simulink library "goose_lib"  (Simulink 8.1)
settings: Solver=ode45  StartTime=0.0  StopTime=10.0  RelTol=1e-3
undefined symbols (not defined in the file or in its folder): CD, relay_iec61850
libraries: rtio_iec61850 x53
settings Model: Creator=re25624  LastModifiedBy=hptb1

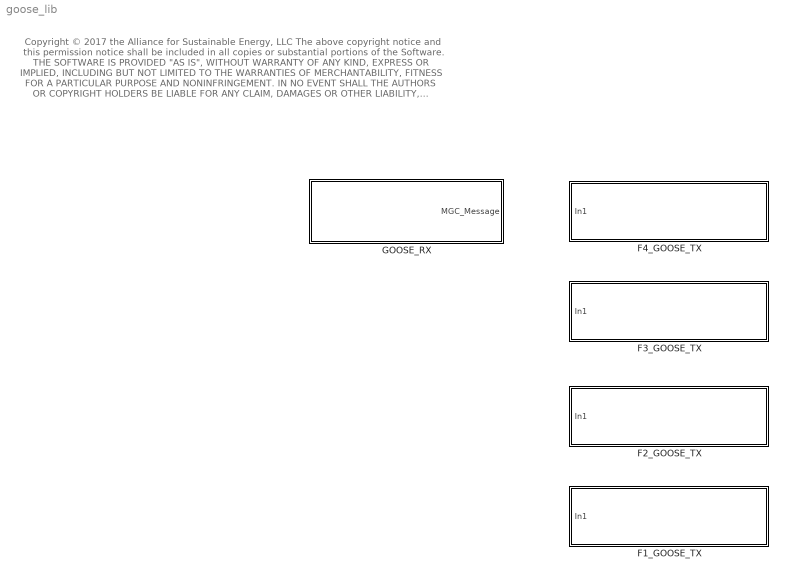
== system goose_lib ==
  note: Copyright © 2017 the Alliance for Sustainable Energy, LLC
      |
      | The above copyright notice and this permission notice shall be included in all copies or substantial portions of the Software.
      |
      | THE SOFTWARE IS PROVIDED "AS IS", WITHOUT WARRANTY OF ANY KIND, EXPRESS OR IMPLIED, INCLUDING
      | BUT NOT LIMITED TO THE WARRANTIES OF MERCHANTABILITY, FITNESS FOR A PARTICULAR PURPOSE AND
      | NONINFRINGEMENT. IN NO EVENT SHALL THE AUTHORS OR COPYRIGHT HOLDERS BE LIABLE FOR ANY CLAIM,
      |  DAMAGES OR OTHER LIABILITY, WHETHER IN AN ACTION OF CONTRACT, TORT OR OTHERWISE, ARISING FROM,
      | OUT OF OR IN CONNECTION WITH THE SOFTWARE OR THE USE OR OTHER DEALINGS IN THE SOFTWARE
  F1_GOOSE_TX : Subsystem
  F2_GOOSE_TX : Subsystem
  F3_GOOSE_TX : Subsystem
  F4_GOOSE_TX : Subsystem
  "GOOSE_RX " : Subsystem

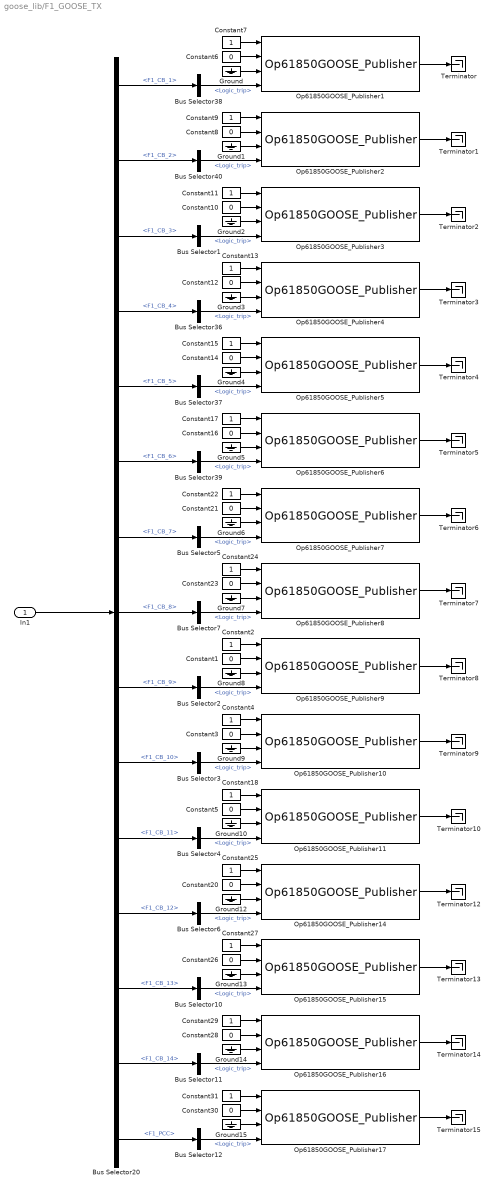
== system goose_lib/F1_GOOSE_TX ==
  In1 : Inport
  Bus Selector{1..7,10..12,36..40} (15 alike) : BusSelector  OutputSignals=Logic_trip
  Bus Selector20 : BusSelector  OutputSignals=F1_CB_1,F1_CB_2,F1_CB_3,F1_CB_4,F1_CB_5,F1_CB_6,F1_CB_7,F1_CB_8,F1_CB_9,F1_CB_10,F1_CB_11,F1_CB_12,F1_CB_13,F1_CB_14,F1_PCC
  Constant{1,3,5..6,8,10,12,14,16,20..21,23,26,28,30} (15 alike) : Constant  Value=0
  Constant{2,4,7,9,11,13,15,17..18,22,24..25,27,29,31} (15 alike) : Constant
  Ground{,1..10,12..15} (15 alike) : Ground
  Op61850GOOSE_Publisher1 : rtio_iec61850/Op61850GOOSE_Publisher  nic_name=eth1  ied_name=CB101  select_scl=off  scl_file=CB101.icd  scl_fullpath=.\relay_iec61850  goose_name=Goose_TRIP1  goose_msgid=0x0101  mac_address=01-0C-CD-01-21-01  vlan_prio=4  vlan_id=000  mintime=25  maxtime=250  gocbref=CB101LDevice1/LLN0$GO$CB_Goose_TRIP1  dataset=CB101LDevice1/LLN0$Goose_TRIP1  goID=Goose_TRIP1  confrev=1  externalClock=off
      settings: AttributesFormatString=%<Name>\nAppId = %<goose_msgid>
  Op61850GOOSE_Publisher10 : rtio_iec61850/Op61850GOOSE_Publisher  nic_name=eth1  ied_name=CB110  select_scl=off  scl_file=CB110.icd  scl_fullpath=.\relay_iec61850  goose_name=Goose_TRIP1  goose_msgid=0x0110  mac_address=01-0C-CD-01-21-10  vlan_prio=4  vlan_id=000  mintime=25  maxtime=250  gocbref=CB110LDevice1/LLN0$GO$CB_Goose_TRIP1  dataset=CB110LDevice1/LLN0$Goose_TRIP1  goID=Goose_TRIP1  confrev=1  externalClock=off
      settings: AttributesFormatString=%<Name>\nAppId = %<goose_msgid>
  Op61850GOOSE_Publisher11 : rtio_iec61850/Op61850GOOSE_Publisher  nic_name=eth1  ied_name=CB111  select_scl=off  scl_file=CB111.icd  scl_fullpath=.\relay_iec61850  goose_name=Goose_TRIP1  goose_msgid=0x0111  mac_address=01-0C-CD-01-21-11  vlan_prio=4  vlan_id=000  mintime=25  maxtime=250  gocbref=CB111LDevice1/LLN0$GO$CB_Goose_TRIP1  dataset=CB111LDevice1/LLN0$Goose_TRIP1  goID=Goose_TRIP1  confrev=1  externalClock=off
      settings: AttributesFormatString=%<Name>\nAppId = %<goose_msgid>
  Op61850GOOSE_Publisher14 : rtio_iec61850/Op61850GOOSE_Publisher  nic_name=eth1  ied_name=CB112  select_scl=off  scl_file=CB112.icd  scl_fullpath=.\relay_iec61850  goose_name=Goose_TRIP1  goose_msgid=0x0112  mac_address=01-0C-CD-01-21-12  vlan_prio=4  vlan_id=000  mintime=25  maxtime=250  gocbref=CB112LDevice1/LLN0$GO$CB_Goose_TRIP1  dataset=CB112LDevice1/LLN0$Goose_TRIP1  goID=Goose_TRIP1  confrev=1  externalClock=off
      settings: AttributesFormatString=%<Name>\nAppId = %<goose_msgid>
  Op61850GOOSE_Publisher15 : rtio_iec61850/Op61850GOOSE_Publisher  nic_name=eth1  ied_name=CB113  select_scl=off  scl_file=CB113.icd  scl_fullpath=.\relay_iec61850  goose_name=Goose_TRIP1  goose_msgid=0x0113  mac_address=01-0C-CD-01-21-13  vlan_prio=4  vlan_id=000  mintime=25  maxtime=250  gocbref=CB113LDevice1/LLN0$GO$CB_Goose_TRIP1  dataset=CB113LDevice1/LLN0$Goose_TRIP1  goID=Goose_TRIP1  confrev=1  externalClock=off
      settings: AttributesFormatString=%<Name>\nAppId = %<goose_msgid>
  Op61850GOOSE_Publisher16 : rtio_iec61850/Op61850GOOSE_Publisher  nic_name=eth1  ied_name=CB114  select_scl=off  scl_file=CB114.icd  scl_fullpath=.\relay_iec61850  goose_name=Goose_TRIP1  goose_msgid=0x0114  mac_address=01-0C-CD-01-21-14  vlan_prio=4  vlan_id=000  mintime=25  maxtime=250  gocbref=CB114LDevice1/LLN0$GO$CB_Goose_TRIP1  dataset=CB114LDevice1/LLN0$Goose_TRIP1  goID=Goose_TRIP1  confrev=1  externalClock=off
      settings: AttributesFormatString=%<Name>\nAppId = %<goose_msgid>
  Op61850GOOSE_Publisher17 : rtio_iec61850/Op61850GOOSE_Publisher  nic_name=eth1  ied_name=CB100  select_scl=off  scl_file=CB100.icd  scl_fullpath=.\relay_iec61850  goose_name=Goose_TRIP1  goose_msgid=0x0100  mac_address=01-0C-CD-01-21-00  vlan_prio=4  vlan_id=000  mintime=25  maxtime=250  gocbref=CB100LDevice1/LLN0$GO$CB_Goose_TRIP1  dataset=CB100LDevice1/LLN0$Goose_TRIP1  goID=Goose_TRIP1  confrev=1  externalClock=off
      settings: AttributesFormatString=%<Name>\nAppId = %<goose_msgid>
  Op61850GOOSE_Publisher2 : rtio_iec61850/Op61850GOOSE_Publisher  nic_name=eth1  ied_name=CB102  select_scl=off  scl_file=CB102.icd  scl_fullpath=.\relay_iec61850  goose_name=Goose_TRIP1  goose_msgid=0x0102  mac_address=01-0C-CD-01-21-02  vlan_prio=4  vlan_id=000  mintime=25  maxtime=250  gocbref=CB102LDevice1/LLN0$GO$CB_Goose_TRIP1  dataset=CB102LDevice1/LLN0$Goose_TRIP1  goID=Goose_TRIP1  confrev=1  externalClock=off
      settings: AttributesFormatString=%<Name>\nAppId = %<goose_msgid>
  Op61850GOOSE_Publisher3 : rtio_iec61850/Op61850GOOSE_Publisher  nic_name=eth1  ied_name=CB103  select_scl=off  scl_file=CB103.icd  scl_fullpath=.\relay_iec61850  goose_name=Goose_TRIP1  goose_msgid=0x0103  mac_address=01-0C-CD-01-21-03  vlan_prio=4  vlan_id=000  mintime=25  maxtime=250  gocbref=CB103LDevice1/LLN0$GO$CB_Goose_TRIP1  dataset=CB103LDevice1/LLN0$Goose_TRIP1  goID=Goose_TRIP1  confrev=1  externalClock=off
      settings: AttributesFormatString=%<Name>\nAppId = %<goose_msgid>
  Op61850GOOSE_Publisher4 : rtio_iec61850/Op61850GOOSE_Publisher  nic_name=eth1  ied_name=CB104  select_scl=off  scl_file=CB104.icd  scl_fullpath=.\relay_iec61850  goose_name=Goose_TRIP1  goose_msgid=0x0104  mac_address=01-0C-CD-01-21-04  vlan_prio=4  vlan_id=000  mintime=25  maxtime=250  gocbref=CB104LDevice1/LLN0$GO$CB_Goose_TRIP1  dataset=CB104LDevice1/LLN0$Goose_TRIP1  goID=Goose_TRIP1  confrev=1  externalClock=off
      settings: AttributesFormatString=%<Name>\nAppId = %<goose_msgid>
  Op61850GOOSE_Publisher5 : rtio_iec61850/Op61850GOOSE_Publisher  nic_name=eth1  ied_name=CB105  select_scl=off  scl_file=CB105.icd  scl_fullpath=.\relay_iec61850  goose_name=Goose_TRIP1  goose_msgid=0x0105  mac_address=01-0C-CD-01-21-05  vlan_prio=4  vlan_id=000  mintime=25  maxtime=250  gocbref=CB105LDevice1/LLN0$GO$CB_Goose_TRIP1  dataset=CB105LDevice1/LLN0$Goose_TRIP1  goID=Goose_TRIP1  confrev=1  externalClock=off
      settings: AttributesFormatString=%<Name>\nAppId = %<goose_msgid>
  Op61850GOOSE_Publisher6 : rtio_iec61850/Op61850GOOSE_Publisher  nic_name=eth1  ied_name=CB106  select_scl=off  scl_file=CB106.icd  scl_fullpath=.\relay_iec61850  goose_name=Goose_TRIP1  goose_msgid=0x0106  mac_address=01-0C-CD-01-21-06  vlan_prio=4  vlan_id=000  mintime=25  maxtime=250  gocbref=CB106LDevice1/LLN0$GO$CB_Goose_TRIP1  dataset=CB106LDevice1/LLN0$Goose_TRIP1  goID=Goose_TRIP1  confrev=1  externalClock=off
      settings: AttributesFormatString=%<Name>\nAppId = %<goose_msgid>
  Op61850GOOSE_Publisher7 : rtio_iec61850/Op61850GOOSE_Publisher  nic_name=eth1  ied_name=CB107  select_scl=off  scl_file=CB107.icd  scl_fullpath=.\relay_iec61850  goose_name=Goose_TRIP1  goose_msgid=0x0107  mac_address=01-0C-CD-01-21-07  vlan_prio=4  vlan_id=000  mintime=25  maxtime=250  gocbref=CB107LDevice1/LLN0$GO$CB_Goose_TRIP1  dataset=CB107LDevice1/LLN0$Goose_TRIP1  goID=Goose_TRIP1  confrev=1  externalClock=off
      settings: AttributesFormatString=%<Name>\nAppId = %<goose_msgid>
  Op61850GOOSE_Publisher8 : rtio_iec61850/Op61850GOOSE_Publisher  nic_name=eth1  ied_name=CB108  select_scl=off  scl_file=CB108.icd  scl_fullpath=.\relay_iec61850  goose_name=Goose_TRIP1  goose_msgid=0x0108  mac_address=01-0C-CD-01-21-08  vlan_prio=4  vlan_id=000  mintime=25  maxtime=250  gocbref=CB108LDevice1/LLN0$GO$CB_Goose_TRIP1  dataset=CB108LDevice1/LLN0$Goose_TRIP1  goID=Goose_TRIP1  confrev=1  externalClock=off
      settings: AttributesFormatString=%<Name>\nAppId = %<goose_msgid>
  Op61850GOOSE_Publisher9 : rtio_iec61850/Op61850GOOSE_Publisher  nic_name=eth1  ied_name=CB109  select_scl=off  scl_file=CB109.icd  scl_fullpath=.\relay_iec61850  goose_name=Goose_TRIP1  goose_msgid=0x0109  mac_address=01-0C-CD-01-21-09  vlan_prio=4  vlan_id=000  mintime=25  maxtime=250  gocbref=CB109LDevice1/LLN0$GO$CB_Goose_TRIP1  dataset=CB109LDevice1/LLN0$Goose_TRIP1  goID=Goose_TRIP1  confrev=1  externalClock=off
      settings: AttributesFormatString=%<Name>\nAppId = %<goose_msgid>
  Terminator{,1..10,12..15} (15 alike) : Terminator
  wires:
  Ground15/1 -> Op61850GOOSE_Publisher17/3
  Constant31/1 -> Op61850GOOSE_Publisher17/1
  Ground13/1 -> Op61850GOOSE_Publisher15/3
  Constant30/1 -> Op61850GOOSE_Publisher17/2
  Bus Selector12/1 -> Op61850GOOSE_Publisher17/4  "<Logic_trip>"
  Bus Selector20/15 -> Bus Selector12/1  "<F1_PCC>"
  Op61850GOOSE_Publisher16/1 -> Terminator14/1
  Ground14/1 -> Op61850GOOSE_Publisher16/3
  Constant26/1 -> Op61850GOOSE_Publisher15/2
  Constant27/1 -> Op61850GOOSE_Publisher15/1
  Bus Selector10/1 -> Op61850GOOSE_Publisher15/4  "<Logic_trip>"
  Bus Selector20/13 -> Bus Selector10/1  "<F1_CB_13>"
  Op61850GOOSE_Publisher14/1 -> Terminator12/1
  Ground12/1 -> Op61850GOOSE_Publisher14/3
  Op61850GOOSE_Publisher15/1 -> Terminator13/1
  Constant28/1 -> Op61850GOOSE_Publisher16/2
  Constant25/1 -> Op61850GOOSE_Publisher14/1
  Constant20/1 -> Op61850GOOSE_Publisher14/2
  Constant29/1 -> Op61850GOOSE_Publisher16/1
  Bus Selector11/1 -> Op61850GOOSE_Publisher16/4  "<Logic_trip>"
  Bus Selector20/14 -> Bus Selector11/1  "<F1_CB_14>"
  Bus Selector20/12 -> Bus Selector6/1  "<F1_CB_12>"
  Bus Selector6/1 -> Op61850GOOSE_Publisher14/4  "<Logic_trip>"
  Op61850GOOSE_Publisher17/1 -> Terminator15/1
  Ground5/1 -> Op61850GOOSE_Publisher6/3
  Constant17/1 -> Op61850GOOSE_Publisher6/1
  Ground3/1 -> Op61850GOOSE_Publisher4/3
  Ground1/1 -> Op61850GOOSE_Publisher2/3
  In1/1 -> Bus Selector20/1
  Constant16/1 -> Op61850GOOSE_Publisher6/2
  Bus Selector39/1 -> Op61850GOOSE_Publisher6/4  "<Logic_trip>"
  Bus Selector20/6 -> Bus Selector39/1  "<F1_CB_6>"
  Op61850GOOSE_Publisher5/1 -> Terminator4/1
  Ground4/1 -> Op61850GOOSE_Publisher5/3
  Constant12/1 -> Op61850GOOSE_Publisher4/2
  Constant13/1 -> Op61850GOOSE_Publisher4/1
  Bus Selector36/1 -> Op61850GOOSE_Publisher4/4  "<Logic_trip>"
  Bus Selector20/4 -> Bus Selector36/1  "<F1_CB_4>"
  Op61850GOOSE_Publisher3/1 -> Terminator2/1
  Constant9/1 -> Op61850GOOSE_Publisher2/1
  Constant8/1 -> Op61850GOOSE_Publisher2/2
  Bus Selector40/1 -> Op61850GOOSE_Publisher2/4  "<Logic_trip>"
  Bus Selector20/2 -> Bus Selector40/1  "<F1_CB_2>"
  Ground2/1 -> Op61850GOOSE_Publisher3/3
  Op61850GOOSE_Publisher1/1 -> Terminator/1
  Op61850GOOSE_Publisher2/1 -> Terminator1/1
  Op61850GOOSE_Publisher4/1 -> Terminator3/1
  Constant14/1 -> Op61850GOOSE_Publisher5/2
  Constant7/1 -> Op61850GOOSE_Publisher1/1
  Ground/1 -> Op61850GOOSE_Publisher1/3
  Constant11/1 -> Op61850GOOSE_Publisher3/1
  Constant10/1 -> Op61850GOOSE_Publisher3/2
  Constant15/1 -> Op61850GOOSE_Publisher5/1
  Bus Selector37/1 -> Op61850GOOSE_Publisher5/4  "<Logic_trip>"
  Bus Selector20/5 -> Bus Selector37/1  "<F1_CB_5>"
  Bus Selector38/1 -> Op61850GOOSE_Publisher1/4  "<Logic_trip>"
  Bus Selector20/1 -> Bus Selector38/1  "<F1_CB_1>"
  Bus Selector20/3 -> Bus Selector1/1  "<F1_CB_3>"
  Bus Selector1/1 -> Op61850GOOSE_Publisher3/4  "<Logic_trip>"
  Constant6/1 -> Op61850GOOSE_Publisher1/2
  Op61850GOOSE_Publisher6/1 -> Terminator5/1
  Ground9/1 -> Op61850GOOSE_Publisher10/3
  Ground7/1 -> Op61850GOOSE_Publisher8/3
  Op61850GOOSE_Publisher11/1 -> Terminator10/1
  Ground10/1 -> Op61850GOOSE_Publisher11/3
  Constant3/1 -> Op61850GOOSE_Publisher10/2
  Constant4/1 -> Op61850GOOSE_Publisher10/1
  Bus Selector3/1 -> Op61850GOOSE_Publisher10/4  "<Logic_trip>"
  Op61850GOOSE_Publisher9/1 -> Terminator8/1
  Constant24/1 -> Op61850GOOSE_Publisher8/1
  Constant23/1 -> Op61850GOOSE_Publisher8/2
  Bus Selector7/1 -> Op61850GOOSE_Publisher8/4  "<Logic_trip>"
  Ground8/1 -> Op61850GOOSE_Publisher9/3
  Op61850GOOSE_Publisher7/1 -> Terminator6/1
  Op61850GOOSE_Publisher8/1 -> Terminator7/1
  Op61850GOOSE_Publisher10/1 -> Terminator9/1
  Constant5/1 -> Op61850GOOSE_Publisher11/2
  Constant22/1 -> Op61850GOOSE_Publisher7/1
  Ground6/1 -> Op61850GOOSE_Publisher7/3
  Constant2/1 -> Op61850GOOSE_Publisher9/1
  Constant1/1 -> Op61850GOOSE_Publisher9/2
  Constant18/1 -> Op61850GOOSE_Publisher11/1
  Bus Selector4/1 -> Op61850GOOSE_Publisher11/4  "<Logic_trip>"
  Bus Selector5/1 -> Op61850GOOSE_Publisher7/4  "<Logic_trip>"
  Bus Selector2/1 -> Op61850GOOSE_Publisher9/4  "<Logic_trip>"
  Constant21/1 -> Op61850GOOSE_Publisher7/2
  Bus Selector20/10 -> Bus Selector3/1  "<F1_CB_10>"
  Bus Selector20/8 -> Bus Selector7/1  "<F1_CB_8>"
  Bus Selector20/11 -> Bus Selector4/1  "<F1_CB_11>"
  Bus Selector20/7 -> Bus Selector5/1  "<F1_CB_7>"
  Bus Selector20/9 -> Bus Selector2/1  "<F1_CB_9>"

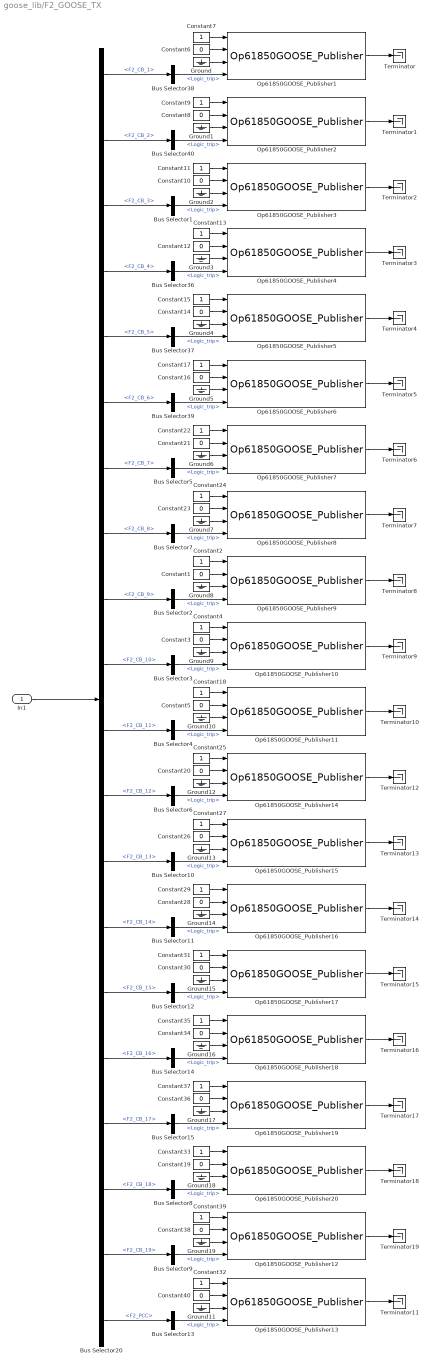
== system goose_lib/F2_GOOSE_TX ==
  In1 : Inport
  Bus Selector{1..15,36..40} (20 alike) : BusSelector  OutputSignals=Logic_trip
  Bus Selector20 : BusSelector  OutputSignals=F2_CB_1,F2_CB_2,F2_CB_3,F2_CB_4,F2_CB_5,F2_CB_6,F2_CB_7,F2_CB_8,F2_CB_9,F2_CB_10,F2_CB_11,F2_CB_12,F2_CB_13,F2_CB_14,F2_CB_15,F2_CB_16,F2_CB_17,F2_CB_18,F2_CB_19,F2_PCC
  Constant{1,3,5..6,8,10,12,14,16,19..21,23,26,28,30,34,36,38,40} (20 alike) : Constant  Value=0
  Constant{2,4,7,9,11,13,15,17..18,22,24..25,27,29,31..33,35,37,39} (20 alike) : Constant
  Ground{,1..19} (20 alike) : Ground
  Op61850GOOSE_Publisher1 : rtio_iec61850/Op61850GOOSE_Publisher  nic_name=eth1  ied_name=CB201  select_scl=off  scl_file=CB201.icd  scl_fullpath=.\relay_iec61850  goose_name=Goose_TRIP1  goose_msgid=0x0201  mac_address=01-0C-CD-01-22-01  vlan_prio=4  vlan_id=000  mintime=25  maxtime=250  gocbref=CB201LDevice1/LLN0$GO$CB_Goose_TRIP1  dataset=CB201LDevice1/LLN0$Goose_TRIP1  goID=Goose_TRIP1  confrev=1  externalClock=off
      settings: AttributesFormatString=%<Name>\nAppId = %<goose_msgid>
  Op61850GOOSE_Publisher10 : rtio_iec61850/Op61850GOOSE_Publisher  nic_name=eth1  ied_name=CB210  select_scl=off  scl_file=CB210.icd  scl_fullpath=.\relay_iec61850  goose_name=Goose_TRIP1  goose_msgid=0x0210  mac_address=01-0C-CD-01-22-10  vlan_prio=4  vlan_id=000  mintime=25  maxtime=250  gocbref=CB210LDevice1/LLN0$GO$CB_Goose_TRIP1  dataset=CB210LDevice1/LLN0$Goose_TRIP1  goID=Goose_TRIP1  confrev=1  externalClock=off
      settings: AttributesFormatString=%<Name>\nAppId = %<goose_msgid>
  Op61850GOOSE_Publisher11 : rtio_iec61850/Op61850GOOSE_Publisher  nic_name=eth1  ied_name=CB211  select_scl=off  scl_file=CB211.icd  scl_fullpath=.\relay_iec61850  goose_name=Goose_TRIP1  goose_msgid=0x0211  mac_address=01-0C-CD-01-22-11  vlan_prio=4  vlan_id=000  mintime=25  maxtime=250  gocbref=CB211LDevice1/LLN0$GO$CB_Goose_TRIP1  dataset=CB211LDevice1/LLN0$Goose_TRIP1  goID=Goose_TRIP1  confrev=1  externalClock=off
      settings: AttributesFormatString=%<Name>\nAppId = %<goose_msgid>
  Op61850GOOSE_Publisher12 : rtio_iec61850/Op61850GOOSE_Publisher  nic_name=eth1  ied_name=CB219  select_scl=off  scl_file=CB219.icd  scl_fullpath=.\relay_iec61850  goose_name=Goose_TRIP1  goose_msgid=0x0219  mac_address=01-0C-CD-01-22-19  vlan_prio=4  vlan_id=000  mintime=25  maxtime=250  gocbref=CB219LDevice1/LLN0$GO$CB_Goose_TRIP1  dataset=CB219LDevice1/LLN0$Goose_TRIP1  goID=Goose_TRIP1  confrev=1  externalClock=off
      settings: AttributesFormatString=%<Name>\nAppId = %<goose_msgid>
  Op61850GOOSE_Publisher13 : rtio_iec61850/Op61850GOOSE_Publisher  nic_name=eth1  ied_name=CB200  select_scl=off  scl_file=CB200.icd  scl_fullpath=.\relay_iec61850  goose_name=Goose_TRIP1  goose_msgid=0x0200  mac_address=01-0C-CD-01-22-00  vlan_prio=4  vlan_id=000  mintime=25  maxtime=250  gocbref=CB200LDevice1/LLN0$GO$CB_Goose_TRIP1  dataset=CB200LDevice1/LLN0$Goose_TRIP1  goID=Goose_TRIP1  confrev=1  externalClock=off
      settings: AttributesFormatString=%<Name>\nAppId = %<goose_msgid>
  Op61850GOOSE_Publisher14 : rtio_iec61850/Op61850GOOSE_Publisher  nic_name=eth1  ied_name=CB212  select_scl=off  scl_file=CB212.icd  scl_fullpath=.\relay_iec61850  goose_name=Goose_TRIP1  goose_msgid=0x0212  mac_address=01-0C-CD-01-22-12  vlan_prio=4  vlan_id=000  mintime=25  maxtime=250  gocbref=CB212LDevice1/LLN0$GO$CB_Goose_TRIP1  dataset=CB212LDevice1/LLN0$Goose_TRIP1  goID=Goose_TRIP1  confrev=1  externalClock=off
      settings: AttributesFormatString=%<Name>\nAppId = %<goose_msgid>
  Op61850GOOSE_Publisher15 : rtio_iec61850/Op61850GOOSE_Publisher  nic_name=eth1  ied_name=CB213  select_scl=off  scl_file=CB213.icd  scl_fullpath=.\relay_iec61850  goose_name=Goose_TRIP1  goose_msgid=0x0213  mac_address=01-0C-CD-01-22-13  vlan_prio=4  vlan_id=000  mintime=25  maxtime=250  gocbref=CB213LDevice1/LLN0$GO$CB_Goose_TRIP1  dataset=CB213LDevice1/LLN0$Goose_TRIP1  goID=Goose_TRIP1  confrev=1  externalClock=off
      settings: AttributesFormatString=%<Name>\nAppId = %<goose_msgid>
  Op61850GOOSE_Publisher16 : rtio_iec61850/Op61850GOOSE_Publisher  nic_name=eth1  ied_name=CB214  select_scl=off  scl_file=CB214.icd  scl_fullpath=.\relay_iec61850  goose_name=Goose_TRIP1  goose_msgid=0x0214  mac_address=01-0C-CD-01-22-14  vlan_prio=4  vlan_id=000  mintime=25  maxtime=250  gocbref=CB214LDevice1/LLN0$GO$CB_Goose_TRIP1  dataset=CB214LDevice1/LLN0$Goose_TRIP1  goID=Goose_TRIP1  confrev=1  externalClock=off
      settings: AttributesFormatString=%<Name>\nAppId = %<goose_msgid>
  Op61850GOOSE_Publisher17 : rtio_iec61850/Op61850GOOSE_Publisher  nic_name=eth1  ied_name=CB215  select_scl=off  scl_file=CB215.icd  scl_fullpath=.\relay_iec61850  goose_name=Goose_TRIP1  goose_msgid=0x0215  mac_address=01-0C-CD-01-22-15  vlan_prio=4  vlan_id=000  mintime=25  maxtime=250  gocbref=CB215LDevice1/LLN0$GO$CB_Goose_TRIP1  dataset=CB215LDevice1/LLN0$Goose_TRIP1  goID=Goose_TRIP1  confrev=1  externalClock=off
      settings: AttributesFormatString=%<Name>\nAppId = %<goose_msgid>
  Op61850GOOSE_Publisher18 : rtio_iec61850/Op61850GOOSE_Publisher  nic_name=eth1  ied_name=CB216  select_scl=off  scl_file=CB216.icd  scl_fullpath=.\relay_iec61850  goose_name=Goose_TRIP1  goose_msgid=0x0216  mac_address=01-0C-CD-01-22-16  vlan_prio=4  vlan_id=000  mintime=25  maxtime=250  gocbref=CB216LDevice1/LLN0$GO$CB_Goose_TRIP1  dataset=CB216LDevice1/LLN0$Goose_TRIP1  goID=Goose_TRIP1  confrev=1  externalClock=off
      settings: AttributesFormatString=%<Name>\nAppId = %<goose_msgid>
  Op61850GOOSE_Publisher19 : rtio_iec61850/Op61850GOOSE_Publisher  nic_name=eth1  ied_name=CB217  select_scl=off  scl_file=CB217.icd  scl_fullpath=.\relay_iec61850  goose_name=Goose_TRIP1  goose_msgid=0x0217  mac_address=01-0C-CD-01-22-17  vlan_prio=4  vlan_id=000  mintime=25  maxtime=250  gocbref=CB217LDevice1/LLN0$GO$CB_Goose_TRIP1  dataset=CB217LDevice1/LLN0$Goose_TRIP1  goID=Goose_TRIP1  confrev=1  externalClock=off
      settings: AttributesFormatString=%<Name>\nAppId = %<goose_msgid>
  Op61850GOOSE_Publisher2 : rtio_iec61850/Op61850GOOSE_Publisher  nic_name=eth1  ied_name=CB202  select_scl=off  scl_file=CB202.icd  scl_fullpath=.\relay_iec61850  goose_name=Goose_TRIP1  goose_msgid=0x0202  mac_address=01-0C-CD-01-22-02  vlan_prio=4  vlan_id=000  mintime=25  maxtime=250  gocbref=CB202LDevice1/LLN0$GO$CB_Goose_TRIP1  dataset=CB202LDevice1/LLN0$Goose_TRIP1  goID=Goose_TRIP1  confrev=1  externalClock=off
      settings: AttributesFormatString=%<Name>\nAppId = %<goose_msgid>
  Op61850GOOSE_Publisher20 : rtio_iec61850/Op61850GOOSE_Publisher  nic_name=eth1  ied_name=CB218  select_scl=off  scl_file=CB218.icd  scl_fullpath=.\relay_iec61850  goose_name=Goose_TRIP1  goose_msgid=0x0218  mac_address=01-0C-CD-01-22-18  vlan_prio=4  vlan_id=000  mintime=25  maxtime=250  gocbref=CB218LDevice1/LLN0$GO$CB_Goose_TRIP1  dataset=CB218LDevice1/LLN0$Goose_TRIP1  goID=Goose_TRIP1  confrev=1  externalClock=off
      settings: AttributesFormatString=%<Name>\nAppId = %<goose_msgid>
  Op61850GOOSE_Publisher3 : rtio_iec61850/Op61850GOOSE_Publisher  nic_name=eth1  ied_name=CB203  select_scl=off  scl_file=CB203.icd  scl_fullpath=.\relay_iec61850  goose_name=Goose_TRIP1  goose_msgid=0x0203  mac_address=01-0C-CD-01-22-03  vlan_prio=4  vlan_id=000  mintime=25  maxtime=250  gocbref=CB203LDevice1/LLN0$GO$CB_Goose_TRIP1  dataset=CB203LDevice1/LLN0$Goose_TRIP1  goID=Goose_TRIP1  confrev=1  externalClock=off
      settings: AttributesFormatString=%<Name>\nAppId = %<goose_msgid>
  Op61850GOOSE_Publisher4 : rtio_iec61850/Op61850GOOSE_Publisher  nic_name=eth1  ied_name=CB204  select_scl=off  scl_file=CB204.icd  scl_fullpath=.\relay_iec61850  goose_name=Goose_TRIP1  goose_msgid=0x0204  mac_address=01-0C-CD-01-22-04  vlan_prio=4  vlan_id=000  mintime=25  maxtime=250  gocbref=CB204LDevice1/LLN0$GO$CB_Goose_TRIP1  dataset=CB204LDevice1/LLN0$Goose_TRIP1  goID=Goose_TRIP1  confrev=1  externalClock=off
      settings: AttributesFormatString=%<Name>\nAppId = %<goose_msgid>
  Op61850GOOSE_Publisher5 : rtio_iec61850/Op61850GOOSE_Publisher  nic_name=eth1  ied_name=CB205  select_scl=off  scl_file=CB205.icd  scl_fullpath=.\relay_iec61850  goose_name=Goose_TRIP1  goose_msgid=0x0205  mac_address=01-0C-CD-01-22-05  vlan_prio=4  vlan_id=000  mintime=25  maxtime=250  gocbref=CB205LDevice1/LLN0$GO$CB_Goose_TRIP1  dataset=CB205LDevice1/LLN0$Goose_TRIP1  goID=Goose_TRIP1  confrev=1  externalClock=off
      settings: AttributesFormatString=%<Name>\nAppId = %<goose_msgid>
  Op61850GOOSE_Publisher6 : rtio_iec61850/Op61850GOOSE_Publisher  nic_name=eth1  ied_name=CB206  select_scl=off  scl_file=CB206.icd  scl_fullpath=.\relay_iec61850  goose_name=Goose_TRIP1  goose_msgid=0x0206  mac_address=01-0C-CD-01-22-06  vlan_prio=4  vlan_id=000  mintime=25  maxtime=250  gocbref=CB206LDevice1/LLN0$GO$CB_Goose_TRIP1  dataset=CB206LDevice1/LLN0$Goose_TRIP1  goID=Goose_TRIP1  confrev=1  externalClock=off
      settings: AttributesFormatString=%<Name>\nAppId = %<goose_msgid>
  Op61850GOOSE_Publisher7 : rtio_iec61850/Op61850GOOSE_Publisher  nic_name=eth1  ied_name=CB207  select_scl=off  scl_file=CB207.icd  scl_fullpath=.\relay_iec61850  goose_name=Goose_TRIP1  goose_msgid=0x0207  mac_address=01-0C-CD-01-22-07  vlan_prio=4  vlan_id=000  mintime=25  maxtime=250  gocbref=CB207LDevice1/LLN0$GO$CB_Goose_TRIP1  dataset=CB207LDevice1/LLN0$Goose_TRIP1  goID=Goose_TRIP1  confrev=1  externalClock=off
      settings: AttributesFormatString=%<Name>\nAppId = %<goose_msgid>
  Op61850GOOSE_Publisher8 : rtio_iec61850/Op61850GOOSE_Publisher  nic_name=eth1  ied_name=CB208  select_scl=off  scl_file=CB208.icd  scl_fullpath=.\relay_iec61850  goose_name=Goose_TRIP1  goose_msgid=0x0208  mac_address=01-0C-CD-01-22-08  vlan_prio=4  vlan_id=000  mintime=25  maxtime=250  gocbref=CB208LDevice1/LLN0$GO$CB_Goose_TRIP1  dataset=CB208LDevice1/LLN0$Goose_TRIP1  goID=Goose_TRIP1  confrev=1  externalClock=off
      settings: AttributesFormatString=%<Name>\nAppId = %<goose_msgid>
  Op61850GOOSE_Publisher9 : rtio_iec61850/Op61850GOOSE_Publisher  nic_name=eth1  ied_name=CB209  select_scl=off  scl_file=CB209.icd  scl_fullpath=.\relay_iec61850  goose_name=Goose_TRIP1  goose_msgid=0x0209  mac_address=01-0C-CD-01-22-09  vlan_prio=4  vlan_id=000  mintime=25  maxtime=250  gocbref=CB209LDevice1/LLN0$GO$CB_Goose_TRIP1  dataset=CB209LDevice1/LLN0$Goose_TRIP1  goID=Goose_TRIP1  confrev=1  externalClock=off
      settings: AttributesFormatString=%<Name>\nAppId = %<goose_msgid>
  Terminator{,1..19} (20 alike) : Terminator
  wires:
  Bus Selector20/9 -> Bus Selector2/1  "<F2_CB_9>"
  Bus Selector20/7 -> Bus Selector5/1  "<F2_CB_7>"
  Bus Selector20/11 -> Bus Selector4/1  "<F2_CB_11>"
  Bus Selector20/8 -> Bus Selector7/1  "<F2_CB_8>"
  Bus Selector20/10 -> Bus Selector3/1  "<F2_CB_10>"
  Constant21/1 -> Op61850GOOSE_Publisher7/2
  Bus Selector2/1 -> Op61850GOOSE_Publisher9/4  "<Logic_trip>"
  Bus Selector5/1 -> Op61850GOOSE_Publisher7/4  "<Logic_trip>"
  Bus Selector4/1 -> Op61850GOOSE_Publisher11/4  "<Logic_trip>"
  Constant18/1 -> Op61850GOOSE_Publisher11/1
  Constant1/1 -> Op61850GOOSE_Publisher9/2
  Constant2/1 -> Op61850GOOSE_Publisher9/1
  Ground6/1 -> Op61850GOOSE_Publisher7/3
  Constant22/1 -> Op61850GOOSE_Publisher7/1
  Constant5/1 -> Op61850GOOSE_Publisher11/2
  Op61850GOOSE_Publisher10/1 -> Terminator9/1
  Op61850GOOSE_Publisher8/1 -> Terminator7/1
  Op61850GOOSE_Publisher7/1 -> Terminator6/1
  Ground8/1 -> Op61850GOOSE_Publisher9/3
  Bus Selector7/1 -> Op61850GOOSE_Publisher8/4  "<Logic_trip>"
  Constant23/1 -> Op61850GOOSE_Publisher8/2
  Constant24/1 -> Op61850GOOSE_Publisher8/1
  Op61850GOOSE_Publisher9/1 -> Terminator8/1
  Bus Selector3/1 -> Op61850GOOSE_Publisher10/4  "<Logic_trip>"
  Constant4/1 -> Op61850GOOSE_Publisher10/1
  Constant3/1 -> Op61850GOOSE_Publisher10/2
  Ground10/1 -> Op61850GOOSE_Publisher11/3
  Op61850GOOSE_Publisher11/1 -> Terminator10/1
  Ground7/1 -> Op61850GOOSE_Publisher8/3
  Ground9/1 -> Op61850GOOSE_Publisher10/3
  Op61850GOOSE_Publisher6/1 -> Terminator5/1
  Constant6/1 -> Op61850GOOSE_Publisher1/2
  Bus Selector1/1 -> Op61850GOOSE_Publisher3/4  "<Logic_trip>"
  Bus Selector20/3 -> Bus Selector1/1  "<F2_CB_3>"
  Bus Selector20/1 -> Bus Selector38/1  "<F2_CB_1>"
  Bus Selector38/1 -> Op61850GOOSE_Publisher1/4  "<Logic_trip>"
  Bus Selector20/5 -> Bus Selector37/1  "<F2_CB_5>"
  Bus Selector37/1 -> Op61850GOOSE_Publisher5/4  "<Logic_trip>"
  Constant15/1 -> Op61850GOOSE_Publisher5/1
  Constant10/1 -> Op61850GOOSE_Publisher3/2
  Constant11/1 -> Op61850GOOSE_Publisher3/1
  Ground/1 -> Op61850GOOSE_Publisher1/3
  Constant7/1 -> Op61850GOOSE_Publisher1/1
  Constant14/1 -> Op61850GOOSE_Publisher5/2
  Op61850GOOSE_Publisher4/1 -> Terminator3/1
  Op61850GOOSE_Publisher2/1 -> Terminator1/1
  Op61850GOOSE_Publisher1/1 -> Terminator/1
  Ground2/1 -> Op61850GOOSE_Publisher3/3
  Bus Selector20/2 -> Bus Selector40/1  "<F2_CB_2>"
  Bus Selector40/1 -> Op61850GOOSE_Publisher2/4  "<Logic_trip>"
  Constant8/1 -> Op61850GOOSE_Publisher2/2
  Constant9/1 -> Op61850GOOSE_Publisher2/1
  Op61850GOOSE_Publisher3/1 -> Terminator2/1
  Bus Selector20/4 -> Bus Selector36/1  "<F2_CB_4>"
  Bus Selector36/1 -> Op61850GOOSE_Publisher4/4  "<Logic_trip>"
  Constant13/1 -> Op61850GOOSE_Publisher4/1
  Constant12/1 -> Op61850GOOSE_Publisher4/2
  Ground4/1 -> Op61850GOOSE_Publisher5/3
  Op61850GOOSE_Publisher5/1 -> Terminator4/1
  Bus Selector20/6 -> Bus Selector39/1  "<F2_CB_6>"
  Bus Selector39/1 -> Op61850GOOSE_Publisher6/4  "<Logic_trip>"
  Constant16/1 -> Op61850GOOSE_Publisher6/2
  In1/1 -> Bus Selector20/1
  Ground1/1 -> Op61850GOOSE_Publisher2/3
  Ground3/1 -> Op61850GOOSE_Publisher4/3
  Constant17/1 -> Op61850GOOSE_Publisher6/1
  Ground5/1 -> Op61850GOOSE_Publisher6/3
  Bus Selector20/18 -> Bus Selector8/1  "<F2_CB_18>"
  Bus Selector20/16 -> Bus Selector14/1  "<F2_CB_16>"
  Bus Selector20/20 -> Bus Selector13/1  "<F2_PCC>"
  Bus Selector20/17 -> Bus Selector15/1  "<F2_CB_17>"
  Bus Selector20/19 -> Bus Selector9/1  "<F2_CB_19>"
  Constant34/1 -> Op61850GOOSE_Publisher18/2
  Bus Selector8/1 -> Op61850GOOSE_Publisher20/4  "<Logic_trip>"
  Bus Selector14/1 -> Op61850GOOSE_Publisher18/4  "<Logic_trip>"
  Bus Selector13/1 -> Op61850GOOSE_Publisher13/4  "<Logic_trip>"
  Constant32/1 -> Op61850GOOSE_Publisher13/1
  Constant19/1 -> Op61850GOOSE_Publisher20/2
  Constant33/1 -> Op61850GOOSE_Publisher20/1
  Ground16/1 -> Op61850GOOSE_Publisher18/3
  Constant35/1 -> Op61850GOOSE_Publisher18/1
  Constant40/1 -> Op61850GOOSE_Publisher13/2
  Op61850GOOSE_Publisher12/1 -> Terminator19/1
  Op61850GOOSE_Publisher19/1 -> Terminator17/1
  Op61850GOOSE_Publisher18/1 -> Terminator16/1
  Ground18/1 -> Op61850GOOSE_Publisher20/3
  Bus Selector15/1 -> Op61850GOOSE_Publisher19/4  "<Logic_trip>"
  Constant36/1 -> Op61850GOOSE_Publisher19/2
  Constant37/1 -> Op61850GOOSE_Publisher19/1
  Op61850GOOSE_Publisher20/1 -> Terminator18/1
  Bus Selector9/1 -> Op61850GOOSE_Publisher12/4  "<Logic_trip>"
  Constant39/1 -> Op61850GOOSE_Publisher12/1
  Constant38/1 -> Op61850GOOSE_Publisher12/2
  Ground11/1 -> Op61850GOOSE_Publisher13/3
  Op61850GOOSE_Publisher13/1 -> Terminator11/1
  Ground17/1 -> Op61850GOOSE_Publisher19/3
  Ground19/1 -> Op61850GOOSE_Publisher12/3
  Op61850GOOSE_Publisher17/1 -> Terminator15/1
  Bus Selector6/1 -> Op61850GOOSE_Publisher14/4  "<Logic_trip>"
  Bus Selector20/12 -> Bus Selector6/1  "<F2_CB_12>"
  Bus Selector20/14 -> Bus Selector11/1  "<F2_CB_14>"
  Bus Selector11/1 -> Op61850GOOSE_Publisher16/4  "<Logic_trip>"
  Constant29/1 -> Op61850GOOSE_Publisher16/1
  Constant20/1 -> Op61850GOOSE_Publisher14/2
  Constant25/1 -> Op61850GOOSE_Publisher14/1
  Constant28/1 -> Op61850GOOSE_Publisher16/2
  Op61850GOOSE_Publisher15/1 -> Terminator13/1
  Ground12/1 -> Op61850GOOSE_Publisher14/3
  Op61850GOOSE_Publisher14/1 -> Terminator12/1
  Bus Selector20/13 -> Bus Selector10/1  "<F2_CB_13>"
  Bus Selector10/1 -> Op61850GOOSE_Publisher15/4  "<Logic_trip>"
  Constant27/1 -> Op61850GOOSE_Publisher15/1
  Constant26/1 -> Op61850GOOSE_Publisher15/2
  Ground14/1 -> Op61850GOOSE_Publisher16/3
  Op61850GOOSE_Publisher16/1 -> Terminator14/1
  Bus Selector20/15 -> Bus Selector12/1  "<F2_CB_15>"
  Bus Selector12/1 -> Op61850GOOSE_Publisher17/4  "<Logic_trip>"
  Constant30/1 -> Op61850GOOSE_Publisher17/2
  Ground13/1 -> Op61850GOOSE_Publisher15/3
  Constant31/1 -> Op61850GOOSE_Publisher17/1
  Ground15/1 -> Op61850GOOSE_Publisher17/3

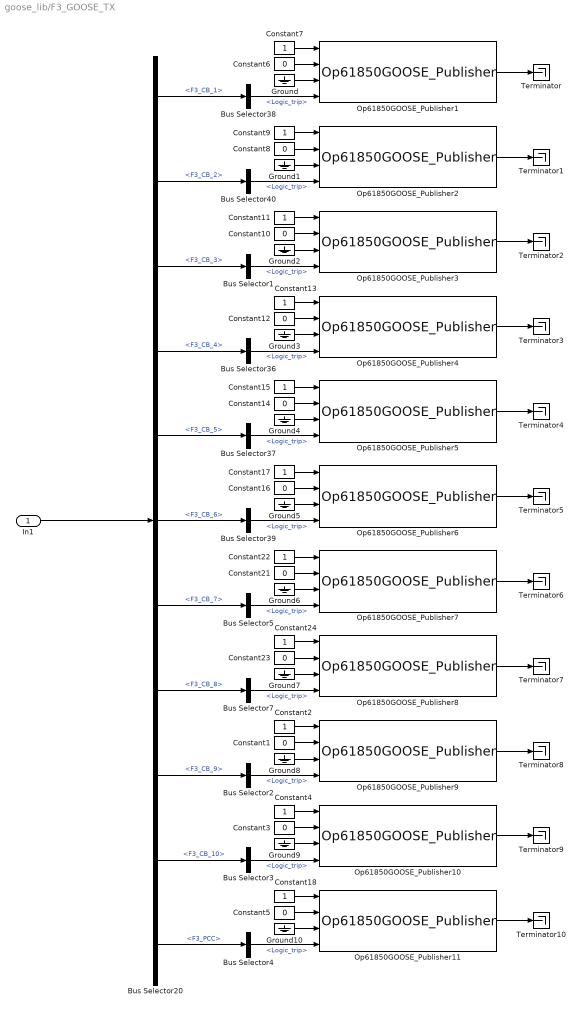
== system goose_lib/F3_GOOSE_TX ==
  In1 : Inport
  Bus Selector{1..5,7,36..40} (11 alike) : BusSelector  OutputSignals=Logic_trip
  Bus Selector20 : BusSelector  OutputSignals=F3_CB_1,F3_CB_2,F3_CB_3,F3_CB_4,F3_CB_5,F3_CB_6,F3_CB_7,F3_CB_8,F3_CB_9,F3_CB_10,F3_PCC
  Constant{1,3,5..6,8,10,12,14,16,21,23} (11 alike) : Constant  Value=0
  Constant{2,4,7,9,11,13,15,17..18,22,24} (11 alike) : Constant
  Ground{,1..10} (11 alike) : Ground
  Op61850GOOSE_Publisher1 : rtio_iec61850/Op61850GOOSE_Publisher  nic_name=eth1  ied_name=CB301  select_scl=off  scl_file=CB301.icd  scl_fullpath=.\relay_iec61850  goose_name=Goose_TRIP1  goose_msgid=0x0301  mac_address=01-0C-CD-01-23-01  vlan_prio=4  vlan_id=000  mintime=25  maxtime=250  gocbref=CB301LDevice1/LLN0$GO$CB_Goose_TRIP1  dataset=CB301LDevice1/LLN0$Goose_TRIP1  goID=Goose_TRIP1  confrev=1  externalClock=off
      settings: AttributesFormatString=%<Name>\nAppId = %<goose_msgid>
  Op61850GOOSE_Publisher10 : rtio_iec61850/Op61850GOOSE_Publisher  nic_name=eth1  ied_name=CB310  select_scl=off  scl_file=CB310.icd  scl_fullpath=.\relay_iec61850  goose_name=Goose_TRIP1  goose_msgid=0x0310  mac_address=01-0C-CD-01-23-10  vlan_prio=4  vlan_id=000  mintime=25  maxtime=250  gocbref=CB310LDevice1/LLN0$GO$CB_Goose_TRIP1  dataset=CB310LDevice1/LLN0$Goose_TRIP1  goID=Goose_TRIP1  confrev=1  externalClock=off
      settings: AttributesFormatString=%<Name>\nAppId = %<goose_msgid>
  Op61850GOOSE_Publisher11 : rtio_iec61850/Op61850GOOSE_Publisher  nic_name=eth1  ied_name=CB300  select_scl=off  scl_file=CB300.icd  scl_fullpath=.\relay_iec61850  goose_name=Goose_TRIP1  goose_msgid=0x0300  mac_address=01-0C-CD-01-23-00  vlan_prio=4  vlan_id=000  mintime=25  maxtime=250  gocbref=CB300LDevice1/LLN0$GO$CB_Goose_TRIP1  dataset=CB300LDevice1/LLN0$Goose_TRIP1  goID=Goose_TRIP1  confrev=1  externalClock=off
      settings: AttributesFormatString=%<Name>\nAppId = %<goose_msgid>
  Op61850GOOSE_Publisher2 : rtio_iec61850/Op61850GOOSE_Publisher  nic_name=eth1  ied_name=CB302  select_scl=off  scl_file=CB302.icd  scl_fullpath=.\relay_iec61850  goose_name=Goose_TRIP1  goose_msgid=0x0302  mac_address=01-0C-CD-01-23-02  vlan_prio=4  vlan_id=000  mintime=25  maxtime=250  gocbref=CB302LDevice1/LLN0$GO$CB_Goose_TRIP1  dataset=CB302LDevice1/LLN0$Goose_TRIP1  goID=Goose_TRIP1  confrev=1  externalClock=off
      settings: AttributesFormatString=%<Name>\nAppId = %<goose_msgid>
  Op61850GOOSE_Publisher3 : rtio_iec61850/Op61850GOOSE_Publisher  nic_name=eth1  ied_name=CB303  select_scl=off  scl_file=CB303.icd  scl_fullpath=.\relay_iec61850  goose_name=Goose_TRIP1  goose_msgid=0x0303  mac_address=01-0C-CD-01-23-03  vlan_prio=4  vlan_id=000  mintime=25  maxtime=250  gocbref=CB303LDevice1/LLN0$GO$CB_Goose_TRIP1  dataset=CB303LDevice1/LLN0$Goose_TRIP1  goID=Goose_TRIP1  confrev=1  externalClock=off
      settings: AttributesFormatString=%<Name>\nAppId = %<goose_msgid>
  Op61850GOOSE_Publisher4 : rtio_iec61850/Op61850GOOSE_Publisher  nic_name=eth1  ied_name=CB304  select_scl=off  scl_file=CB304.icd  scl_fullpath=.\relay_iec61850  goose_name=Goose_TRIP1  goose_msgid=0x0304  mac_address=01-0C-CD-01-23-04  vlan_prio=4  vlan_id=000  mintime=25  maxtime=250  gocbref=CB304LDevice1/LLN0$GO$CB_Goose_TRIP1  dataset=CB304LDevice1/LLN0$Goose_TRIP1  goID=Goose_TRIP1  confrev=1  externalClock=off
      settings: AttributesFormatString=%<Name>\nAppId = %<goose_msgid>
  Op61850GOOSE_Publisher5 : rtio_iec61850/Op61850GOOSE_Publisher  nic_name=eth1  ied_name=CB305  select_scl=off  scl_file=CB305.icd  scl_fullpath=.\relay_iec61850  goose_name=Goose_TRIP1  goose_msgid=0x0305  mac_address=01-0C-CD-01-23-05  vlan_prio=4  vlan_id=000  mintime=25  maxtime=250  gocbref=CB305LDevice1/LLN0$GO$CB_Goose_TRIP1  dataset=CB305LDevice1/LLN0$Goose_TRIP1  goID=Goose_TRIP1  confrev=1  externalClock=off
      settings: AttributesFormatString=%<Name>\nAppId = %<goose_msgid>
  Op61850GOOSE_Publisher6 : rtio_iec61850/Op61850GOOSE_Publisher  nic_name=eth1  ied_name=CB306  select_scl=off  scl_file=CB306.icd  scl_fullpath=.\relay_iec61850  goose_name=Goose_TRIP1  goose_msgid=0x0306  mac_address=01-0C-CD-01-23-06  vlan_prio=4  vlan_id=000  mintime=25  maxtime=250  gocbref=CB306LDevice1/LLN0$GO$CB_Goose_TRIP1  dataset=CB306LDevice1/LLN0$Goose_TRIP1  goID=Goose_TRIP1  confrev=1  externalClock=off
      settings: AttributesFormatString=%<Name>\nAppId = %<goose_msgid>
  Op61850GOOSE_Publisher7 : rtio_iec61850/Op61850GOOSE_Publisher  nic_name=eth1  ied_name=CB307  select_scl=off  scl_file=CB307.icd  scl_fullpath=.\relay_iec61850  goose_name=Goose_TRIP1  goose_msgid=0x0307  mac_address=01-0C-CD-01-23-07  vlan_prio=4  vlan_id=000  mintime=25  maxtime=250  gocbref=CB307LDevice1/LLN0$GO$CB_Goose_TRIP1  dataset=CB307LDevice1/LLN0$Goose_TRIP1  goID=Goose_TRIP1  confrev=1  externalClock=off
      settings: AttributesFormatString=%<Name>\nAppId = %<goose_msgid>
  Op61850GOOSE_Publisher8 : rtio_iec61850/Op61850GOOSE_Publisher  nic_name=eth1  ied_name=CB308  select_scl=off  scl_file=CB308.icd  scl_fullpath=.\relay_iec61850  goose_name=Goose_TRIP1  goose_msgid=0x0308  mac_address=01-0C-CD-01-23-08  vlan_prio=4  vlan_id=000  mintime=25  maxtime=250  gocbref=CB308LDevice1/LLN0$GO$CB_Goose_TRIP1  dataset=CB308LDevice1/LLN0$Goose_TRIP1  goID=Goose_TRIP1  confrev=1  externalClock=off
      settings: AttributesFormatString=%<Name>\nAppId = %<goose_msgid>
  Op61850GOOSE_Publisher9 : rtio_iec61850/Op61850GOOSE_Publisher  nic_name=eth1  ied_name=CB309  select_scl=off  scl_file=CB309.icd  scl_fullpath=.\relay_iec61850  goose_name=Goose_TRIP1  goose_msgid=0x0309  mac_address=01-0C-CD-01-23-09  vlan_prio=4  vlan_id=000  mintime=25  maxtime=250  gocbref=CB309LDevice1/LLN0$GO$CB_Goose_TRIP1  dataset=CB309LDevice1/LLN0$Goose_TRIP1  goID=Goose_TRIP1  confrev=1  externalClock=off
      settings: AttributesFormatString=%<Name>\nAppId = %<goose_msgid>
  Terminator{,1..10} (11 alike) : Terminator
  wires:
  Ground5/1 -> Op61850GOOSE_Publisher6/3
  Constant17/1 -> Op61850GOOSE_Publisher6/1
  Ground3/1 -> Op61850GOOSE_Publisher4/3
  Ground1/1 -> Op61850GOOSE_Publisher2/3
  In1/1 -> Bus Selector20/1
  Constant16/1 -> Op61850GOOSE_Publisher6/2
  Bus Selector39/1 -> Op61850GOOSE_Publisher6/4  "<Logic_trip>"
  Bus Selector20/6 -> Bus Selector39/1  "<F3_CB_6>"
  Op61850GOOSE_Publisher5/1 -> Terminator4/1
  Ground4/1 -> Op61850GOOSE_Publisher5/3
  Constant12/1 -> Op61850GOOSE_Publisher4/2
  Constant13/1 -> Op61850GOOSE_Publisher4/1
  Bus Selector36/1 -> Op61850GOOSE_Publisher4/4  "<Logic_trip>"
  Bus Selector20/4 -> Bus Selector36/1  "<F3_CB_4>"
  Op61850GOOSE_Publisher3/1 -> Terminator2/1
  Constant9/1 -> Op61850GOOSE_Publisher2/1
  Constant8/1 -> Op61850GOOSE_Publisher2/2
  Bus Selector40/1 -> Op61850GOOSE_Publisher2/4  "<Logic_trip>"
  Bus Selector20/2 -> Bus Selector40/1  "<F3_CB_2>"
  Ground2/1 -> Op61850GOOSE_Publisher3/3
  Op61850GOOSE_Publisher1/1 -> Terminator/1
  Op61850GOOSE_Publisher2/1 -> Terminator1/1
  Op61850GOOSE_Publisher4/1 -> Terminator3/1
  Constant14/1 -> Op61850GOOSE_Publisher5/2
  Constant7/1 -> Op61850GOOSE_Publisher1/1
  Ground/1 -> Op61850GOOSE_Publisher1/3
  Constant11/1 -> Op61850GOOSE_Publisher3/1
  Constant10/1 -> Op61850GOOSE_Publisher3/2
  Constant15/1 -> Op61850GOOSE_Publisher5/1
  Bus Selector37/1 -> Op61850GOOSE_Publisher5/4  "<Logic_trip>"
  Bus Selector20/5 -> Bus Selector37/1  "<F3_CB_5>"
  Bus Selector38/1 -> Op61850GOOSE_Publisher1/4  "<Logic_trip>"
  Bus Selector20/1 -> Bus Selector38/1  "<F3_CB_1>"
  Bus Selector20/3 -> Bus Selector1/1  "<F3_CB_3>"
  Bus Selector1/1 -> Op61850GOOSE_Publisher3/4  "<Logic_trip>"
  Constant6/1 -> Op61850GOOSE_Publisher1/2
  Op61850GOOSE_Publisher6/1 -> Terminator5/1
  Ground9/1 -> Op61850GOOSE_Publisher10/3
  Ground7/1 -> Op61850GOOSE_Publisher8/3
  Op61850GOOSE_Publisher11/1 -> Terminator10/1
  Ground10/1 -> Op61850GOOSE_Publisher11/3
  Constant3/1 -> Op61850GOOSE_Publisher10/2
  Constant4/1 -> Op61850GOOSE_Publisher10/1
  Bus Selector3/1 -> Op61850GOOSE_Publisher10/4  "<Logic_trip>"
  Op61850GOOSE_Publisher9/1 -> Terminator8/1
  Constant24/1 -> Op61850GOOSE_Publisher8/1
  Constant23/1 -> Op61850GOOSE_Publisher8/2
  Bus Selector7/1 -> Op61850GOOSE_Publisher8/4  "<Logic_trip>"
  Ground8/1 -> Op61850GOOSE_Publisher9/3
  Op61850GOOSE_Publisher7/1 -> Terminator6/1
  Op61850GOOSE_Publisher8/1 -> Terminator7/1
  Op61850GOOSE_Publisher10/1 -> Terminator9/1
  Constant5/1 -> Op61850GOOSE_Publisher11/2
  Constant22/1 -> Op61850GOOSE_Publisher7/1
  Ground6/1 -> Op61850GOOSE_Publisher7/3
  Constant2/1 -> Op61850GOOSE_Publisher9/1
  Constant1/1 -> Op61850GOOSE_Publisher9/2
  Constant18/1 -> Op61850GOOSE_Publisher11/1
  Bus Selector4/1 -> Op61850GOOSE_Publisher11/4  "<Logic_trip>"
  Bus Selector5/1 -> Op61850GOOSE_Publisher7/4  "<Logic_trip>"
  Bus Selector2/1 -> Op61850GOOSE_Publisher9/4  "<Logic_trip>"
  Constant21/1 -> Op61850GOOSE_Publisher7/2
  Bus Selector20/10 -> Bus Selector3/1  "<F3_CB_10>"
  Bus Selector20/8 -> Bus Selector7/1  "<F3_CB_8>"
  Bus Selector20/11 -> Bus Selector4/1  "<F3_PCC>"
  Bus Selector20/7 -> Bus Selector5/1  "<F3_CB_7>"
  Bus Selector20/9 -> Bus Selector2/1  "<F3_CB_9>"

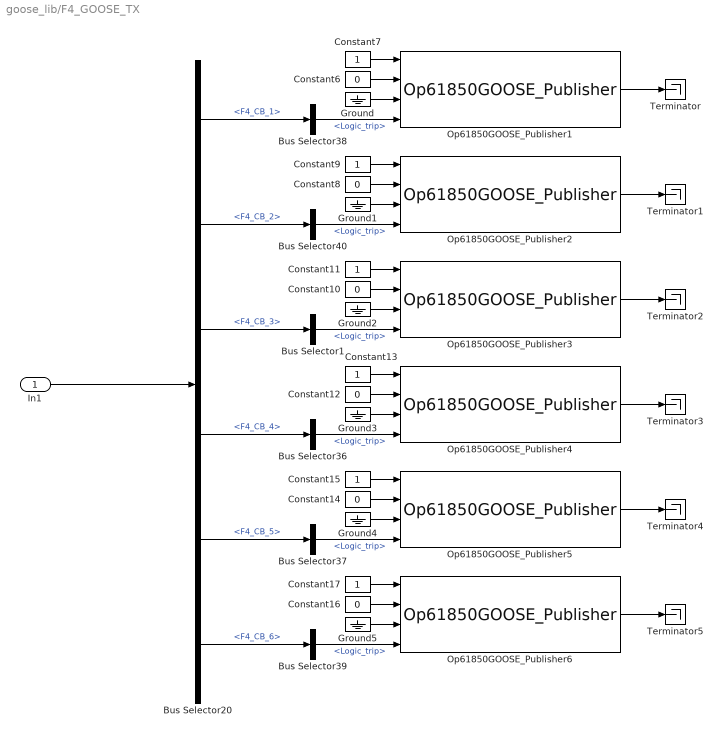
== system goose_lib/F4_GOOSE_TX ==
  In1 : Inport
  Bus Selector{1,36..40} (6 alike) : BusSelector  OutputSignals=Logic_trip
  Bus Selector20 : BusSelector  OutputSignals=F4_CB_1,F4_CB_2,F4_CB_3,F4_CB_4,F4_CB_5,F4_CB_6
  Constant{6,8,10,12,14,16} (6 alike) : Constant  Value=0
  Constant{7,9,11,13,15,17} (6 alike) : Constant
  Ground{,1..5} (6 alike) : Ground
  Op61850GOOSE_Publisher1 : rtio_iec61850/Op61850GOOSE_Publisher  nic_name=eth1  ied_name=CB401  select_scl=off  scl_file=CB401.icd  scl_fullpath=.\relay_iec61850  goose_name=Goose_TRIP1  goose_msgid=0x0401  mac_address=01-0C-CD-01-24-01  vlan_prio=4  vlan_id=000  mintime=25  maxtime=250  gocbref=CB401LDevice1/LLN0$GO$CB_Goose_TRIP1  dataset=CB401LDevice1/LLN0$Goose_TRIP1  goID=Goose_TRIP1  confrev=1  externalClock=off
      settings: AttributesFormatString=%<Name>\nAppId = %<goose_msgid>
  Op61850GOOSE_Publisher2 : rtio_iec61850/Op61850GOOSE_Publisher  nic_name=eth1  ied_name=CB402  select_scl=off  scl_file=CB402.icd  scl_fullpath=.\relay_iec61850  goose_name=Goose_TRIP1  goose_msgid=0x0402  mac_address=01-0C-CD-01-24-02  vlan_prio=4  vlan_id=000  mintime=25  maxtime=250  gocbref=CB402LDevice1/LLN0$GO$CB_Goose_TRIP1  dataset=CB402LDevice1/LLN0$Goose_TRIP1  goID=Goose_TRIP1  confrev=1  externalClock=off
      settings: AttributesFormatString=%<Name>\nAppId = %<goose_msgid>
  Op61850GOOSE_Publisher3 : rtio_iec61850/Op61850GOOSE_Publisher  nic_name=eth1  ied_name=CB403  select_scl=off  scl_file=CB403.icd  scl_fullpath=.\relay_iec61850  goose_name=Goose_TRIP1  goose_msgid=0x0403  mac_address=01-0C-CD-01-24-03  vlan_prio=4  vlan_id=000  mintime=25  maxtime=250  gocbref=CB403LDevice1/LLN0$GO$CB_Goose_TRIP1  dataset=CB403LDevice1/LLN0$Goose_TRIP1  goID=Goose_TRIP1  confrev=1  externalClock=off
      settings: AttributesFormatString=%<Name>\nAppId = %<goose_msgid>
  Op61850GOOSE_Publisher4 : rtio_iec61850/Op61850GOOSE_Publisher  nic_name=eth1  ied_name=CB404  select_scl=off  scl_file=CB404.icd  scl_fullpath=.\relay_iec61850  goose_name=Goose_TRIP1  goose_msgid=0x0404  mac_address=01-0C-CD-01-24-04  vlan_prio=4  vlan_id=000  mintime=25  maxtime=250  gocbref=CB404LDevice1/LLN0$GO$CB_Goose_TRIP1  dataset=CB404LDevice1/LLN0$Goose_TRIP1  goID=Goose_TRIP1  confrev=1  externalClock=off
      settings: AttributesFormatString=%<Name>\nAppId = %<goose_msgid>
  Op61850GOOSE_Publisher5 : rtio_iec61850/Op61850GOOSE_Publisher  nic_name=eth1  ied_name=CB405  select_scl=off  scl_file=CB405.icd  scl_fullpath=.\relay_iec61850  goose_name=Goose_TRIP1  goose_msgid=0x0405  mac_address=01-0C-CD-01-24-05  vlan_prio=4  vlan_id=000  mintime=25  maxtime=250  gocbref=CB405LDevice1/LLN0$GO$CB_Goose_TRIP1  dataset=CB405LDevice1/LLN0$Goose_TRIP1  goID=Goose_TRIP1  confrev=1  externalClock=off
      settings: AttributesFormatString=%<Name>\nAppId = %<goose_msgid>
  Op61850GOOSE_Publisher6 : rtio_iec61850/Op61850GOOSE_Publisher  nic_name=eth1  ied_name=CB406  select_scl=off  scl_file=CB406.icd  scl_fullpath=.\relay_iec61850  goose_name=Goose_TRIP1  goose_msgid=0x0406  mac_address=01-0C-CD-01-24-06  vlan_prio=4  vlan_id=000  mintime=25  maxtime=250  gocbref=CB406LDevice1/LLN0$GO$CB_Goose_TRIP1  dataset=CB406LDevice1/LLN0$Goose_TRIP1  goID=Goose_TRIP1  confrev=1  externalClock=off
      settings: AttributesFormatString=%<Name>\nAppId = %<goose_msgid>
  Terminator{,1..5} (6 alike) : Terminator
  wires:
  Op61850GOOSE_Publisher6/1 -> Terminator5/1
  Constant6/1 -> Op61850GOOSE_Publisher1/2
  Bus Selector1/1 -> Op61850GOOSE_Publisher3/4  "<Logic_trip>"
  Bus Selector20/3 -> Bus Selector1/1  "<F4_CB_3>"
  Bus Selector20/1 -> Bus Selector38/1  "<F4_CB_1>"
  Bus Selector38/1 -> Op61850GOOSE_Publisher1/4  "<Logic_trip>"
  Bus Selector20/5 -> Bus Selector37/1  "<F4_CB_5>"
  Bus Selector37/1 -> Op61850GOOSE_Publisher5/4  "<Logic_trip>"
  Constant15/1 -> Op61850GOOSE_Publisher5/1
  Constant10/1 -> Op61850GOOSE_Publisher3/2
  Constant11/1 -> Op61850GOOSE_Publisher3/1
  Ground/1 -> Op61850GOOSE_Publisher1/3
  Constant7/1 -> Op61850GOOSE_Publisher1/1
  Constant14/1 -> Op61850GOOSE_Publisher5/2
  Op61850GOOSE_Publisher4/1 -> Terminator3/1
  Op61850GOOSE_Publisher2/1 -> Terminator1/1
  Op61850GOOSE_Publisher1/1 -> Terminator/1
  Ground2/1 -> Op61850GOOSE_Publisher3/3
  Bus Selector20/2 -> Bus Selector40/1  "<F4_CB_2>"
  Bus Selector40/1 -> Op61850GOOSE_Publisher2/4  "<Logic_trip>"
  Constant8/1 -> Op61850GOOSE_Publisher2/2
  Constant9/1 -> Op61850GOOSE_Publisher2/1
  Op61850GOOSE_Publisher3/1 -> Terminator2/1
  Bus Selector20/4 -> Bus Selector36/1  "<F4_CB_4>"
  Bus Selector36/1 -> Op61850GOOSE_Publisher4/4  "<Logic_trip>"
  Constant13/1 -> Op61850GOOSE_Publisher4/1
  Constant12/1 -> Op61850GOOSE_Publisher4/2
  Ground4/1 -> Op61850GOOSE_Publisher5/3
  Op61850GOOSE_Publisher5/1 -> Terminator4/1
  Bus Selector20/6 -> Bus Selector39/1  "<F4_CB_6>"
  Bus Selector39/1 -> Op61850GOOSE_Publisher6/4  "<Logic_trip>"
  Constant16/1 -> Op61850GOOSE_Publisher6/2
  In1/1 -> Bus Selector20/1
  Ground1/1 -> Op61850GOOSE_Publisher2/3
  Ground3/1 -> Op61850GOOSE_Publisher4/3
  Constant17/1 -> Op61850GOOSE_Publisher6/1
  Ground5/1 -> Op61850GOOSE_Publisher6/3

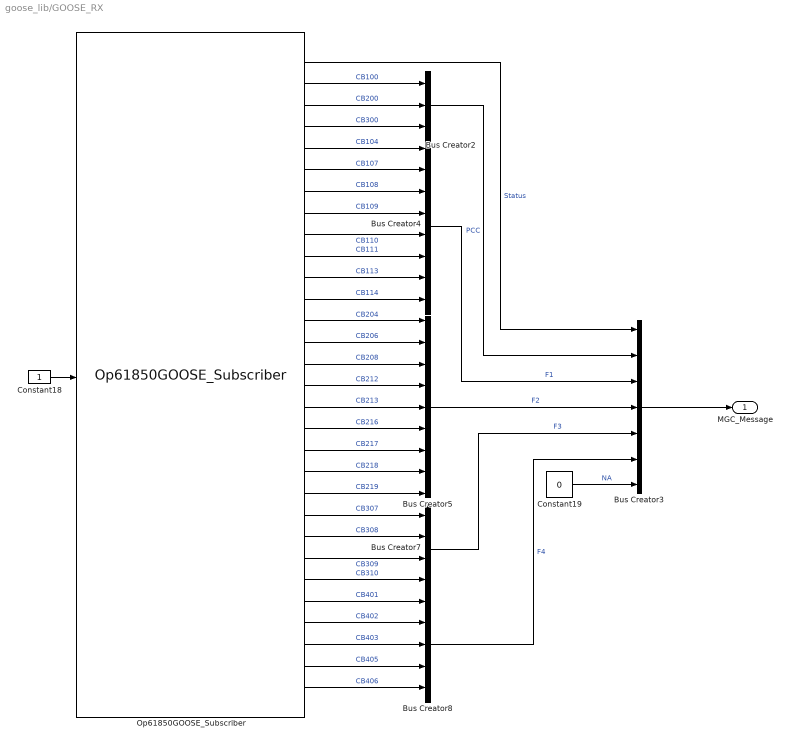
== system goose_lib/GOOSE_RX  ==
  Bus Creator2 : BusCreator  Inputs=3
  Bus Creator3 : BusCreator  Inputs=7
  Bus Creator4 : BusCreator  Inputs=8
  Bus Creator5 : BusCreator  Inputs=9
  Bus Creator7 : BusCreator
  Bus Creator8 : BusCreator  Inputs=5
  Constant18 : Constant
  Constant19 : Constant  Value=0
  Op61850GOOSE_Subscriber : rtio_iec61850/Op61850GOOSE_Subscriber  nic_name=eth1  ied_name=MGC  select_scl=off  scl_file=MGC.ICD  scl_fullpath=.\relay_iec61850  goose_name=Goose_MGCcmd  goose_msgid=0x0001  mac_address=01-0C-CD-01-28-60
      settings: AttributesFormatString=%<Name>\nAppId = %<goose_msgid>
  MGC_Message : Outport
  wires:
  Op61850GOOSE_Subscriber/26 -> Bus Creator8/1  "CB401"
  Op61850GOOSE_Subscriber/27 -> Bus Creator8/2  "CB402"
  Op61850GOOSE_Subscriber/29 -> Bus Creator8/4  "CB405"
  Constant19/1 -> Bus Creator3/7  "NA"
  Op61850GOOSE_Subscriber/22 -> Bus Creator7/1  "CB307"
  Op61850GOOSE_Subscriber/23 -> Bus Creator7/2  "CB308"
  Op61850GOOSE_Subscriber/24 -> Bus Creator7/3  "CB309"
  Op61850GOOSE_Subscriber/25 -> Bus Creator7/4  "CB310"
  Bus Creator7/1 -> Bus Creator3/5  "F3"
  Op61850GOOSE_Subscriber/28 -> Bus Creator8/3  "CB403"
  Op61850GOOSE_Subscriber/30 -> Bus Creator8/5  "CB406"
  Bus Creator8/1 -> Bus Creator3/6  "F4"
  Bus Creator5/1 -> Bus Creator3/4  "F2"
  Op61850GOOSE_Subscriber/14 -> Bus Creator5/2  "CB206"
  Op61850GOOSE_Subscriber/16 -> Bus Creator5/4  "CB212"
  Op61850GOOSE_Subscriber/13 -> Bus Creator5/1  "CB204"
  Op61850GOOSE_Subscriber/15 -> Bus Creator5/3  "CB208"
  Op61850GOOSE_Subscriber/20 -> Bus Creator5/8  "CB218"
  Op61850GOOSE_Subscriber/17 -> Bus Creator5/5  "CB213"
  Op61850GOOSE_Subscriber/19 -> Bus Creator5/7  "CB217"
  Op61850GOOSE_Subscriber/18 -> Bus Creator5/6  "CB216"
  Op61850GOOSE_Subscriber/21 -> Bus Creator5/9  "CB219"
  Bus Creator4/1 -> Bus Creator3/3  "F1"
  Op61850GOOSE_Subscriber/12 -> Bus Creator4/8  "CB114"
  Op61850GOOSE_Subscriber/11 -> Bus Creator4/7  "CB113"
  Op61850GOOSE_Subscriber/10 -> Bus Creator4/6  "CB111"
  Op61850GOOSE_Subscriber/5 -> Bus Creator4/1  "CB104"
  Op61850GOOSE_Subscriber/9 -> Bus Creator4/5  "CB110"
  Op61850GOOSE_Subscriber/6 -> Bus Creator4/2  "CB107"
  Op61850GOOSE_Subscriber/8 -> Bus Creator4/4  "CB109"
  Op61850GOOSE_Subscriber/7 -> Bus Creator4/3  "CB108"
  Bus Creator2/1 -> Bus Creator3/2  "PCC"
  Op61850GOOSE_Subscriber/4 -> Bus Creator2/3  "CB300"
  Op61850GOOSE_Subscriber/3 -> Bus Creator2/2  "CB200"
  Op61850GOOSE_Subscriber/2 -> Bus Creator2/1  "CB100"
  Bus Creator3/1 -> MGC_Message/1
  Op61850GOOSE_Subscriber/1 -> Bus Creator3/1  "Status"
  Constant18/1 -> Op61850GOOSE_Subscriber/1
